simulink model "prob3"  (R2020a)
settings: Solver=ode45  StartTime=0.0  StopTime=120  RelTol=1e-3
values from neighbouring files (symbols this model uses):
  ki = 40.0    [data.sldd]    (also in para3.m = 40)
  kp = 800.0    [data.sldd]    (also in para3.m = 800)
settings Model: DataDictionary=data.sldd  Creator=vijay  LastModifiedBy=vijay

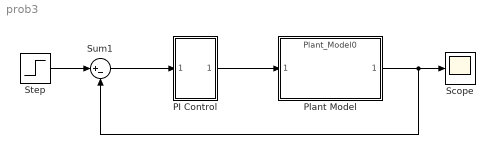
== system prob3 ==
  PI Control : Subsystem
  Plant Model : ModelReference  ModelNameDialog=Plant_Model0  SimulationMode=Normal  ModelReferenceVersion=1.5
  Scope : Scope
  Step : Step  Time=0  After=u  SampleTime=0
  Sum1 : Sum  Inputs=|+-
  wires:
  Plant Model/1 -> Sum1/2, Scope/1
  Step/1 -> Sum1/1
  Sum1/1 -> PI Control/1(In1)
  PI Control/1(Out1) -> Plant Model/1

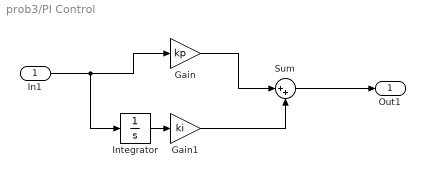
== system prob3/PI Control ==
  In1 : Inport
  Gain : Gain  Gain=kp
  Gain1 : Gain  Gain=ki
  Integrator : Integrator
  Sum : Sum  Inputs=|++
  Out1 : Outport
  wires:
  Gain1/1 -> Sum/2
  Integrator/1 -> Gain1/1
  Gain/1 -> Sum/1
  In1/1 -> Integrator/1, Gain/1
  Sum/1 -> Out1/1
